simulink model "SimulateHVDC"  (R2024b)
settings: Solver=VariableStepAuto  StartTime=0.0  StopTime=Tf  FixedStep=Ti  MaxStep=Ti  RelTol=1e-6
InitFcn:
  | sim_initHVDC
StartFcn:
  | sim_initHVDC
undefined symbols (not defined in the file): CCMPC, CEMPC, DiscIntNeverNeededParam, GCC, M2C, PCC, plecs, PLL, RFT, TEB, Ti, Ts_cc, Ts_ce, Xmax, Ymax
libraries: slpidlib x5, dspstat3 x5, simulink_extras x2, spsdq0toAlphaBetaZeroLib x2, spsAlphaBetaZerotodq0Lib x2, spsabctoAlphaBetaZeroLib x2, rllib x1, deeplib x1, embmathops x1, spsabctodq0Lib x1, spsAlphaBetaZerotoabcLib x1
(part 1 of 2)
settings Model: Creator=Pablo  LastModifiedBy=Ingeniería Eléctrica
settings SolverCC: InitialStep=Ti/10  MinimalZcImpactIntegration=on

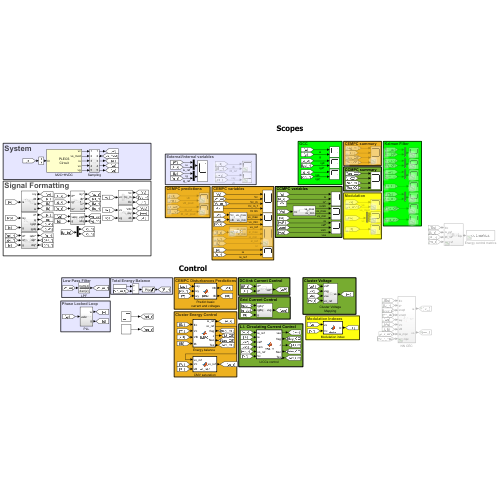
[thumbnail: Simulink's stored preview of the top-level diagram]
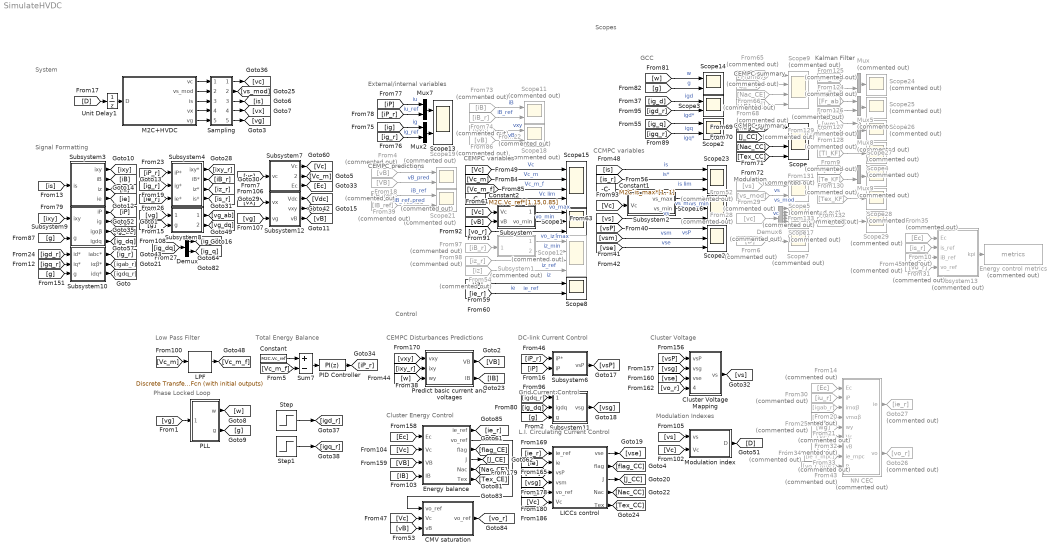
== system SimulateHVDC ==
  note: Control
  note: System
  note: Signal Formatting
  note: CCMPC summary
  note: DC-link Current Control
  note: Modulation Indexes
  note: CEMPC variables
  note: Total Energy Balance
  note: Modulation
  note: External/internal variables
  note: GCC
  note: CCMPC variables
  note: Kalman Filter
  note: CEMPC predictions
  note: CEMPC summary
  note: Low Pass Filter
  note: Cluster Energy Control
  note: CEMPC Disturbances Predictions
  note: Scopes
  note: Grid Current Control
  note: L.I. Circulating Current Control
  note: Cluster Voltage
  note: Phase Locked Loop
  CMV saturation : MATLAB Function  TreatAsAtomicUnit=on  SystemSampleTime=Ts_cc
  Cluster Voltage Mapping : Subsystem
  Constant : Constant  Value=M2C.Vc_ref  SampleTime=Ts_ce
  Constant1 : Constant  Value=M2C.is_max*[1,-1]  SampleTime=Ts_cc
  Constant2 : Constant  Value=M2C.Vc_ref*[1.15,0.85]  SampleTime=Ts_cc
  Demux : Demux  Outputs=2
  Demux6 : Demux  Commented=on  Outputs=M2C.m
  Energy balance : MATLAB Function  TreatAsAtomicUnit=on  SystemSampleTime=CEMPC.Ts
  Energy control metrics : ToWorkspace  Commented=on  VariableName=metrics  SaveFormat=Timeseries  SampleTime=-1
  From10 : From  Commented=on  GotoTag=is_r
  From124 : From  Commented=on  GotoTag=im_ab
  From125 : From  Commented=on  GotoTag=im_KF
  From126 : From  Commented=on  GotoTag=Fr_ab
  From127 : From  Commented=on  GotoTag=Fr_KF
  From128 : From  Commented=on  GotoTag=wm
  From129 : From  Commented=on  GotoTag=wm_KF
  From130 : From  Commented=on  GotoTag=Te
  From131 : From  Commented=on  GotoTag=Te_KF
  From132 : From  Commented=on  GotoTag=Tex_KF
  From133 : From  Commented=on  GotoTag=NIS_KF
  From14 : From  Commented=on  GotoTag=Ec
  From18 : From  Commented=on  GotoTag=VB
  From20 : From  Commented=on  GotoTag=igab_r
  From21 : From  Commented=on  GotoTag=vm_ab
  From22 : From  Commented=on  GotoTag=vB
  From25 : From  Commented=on  GotoTag=wg
  From28 : From  Commented=on  GotoTag=vc
  From29 : From  Commented=on  GotoTag=vs
  From30 : From  Commented=on  GotoTag=iu_r
  From31 : From  Commented=on  GotoTag=iB_r
  From32 : From  Commented=on  GotoTag=Vc
  From33 : From  Commented=on  GotoTag=vB
  From34 : From  Commented=on  GotoTag=ie_r_mpc
  From35 : From  Commented=on  GotoTag=Ec
  From36 : From  Commented=on  GotoTag=IB_ref
  From39 : From  Commented=on  GotoTag=iB_ref
  From4 : From  Commented=on  GotoTag=vB
  From43 : From  Commented=on  GotoTag=vo_r_mpc
  From45 : From  Commented=on  GotoTag=vo_r
  From52 : From  Commented=on  GotoTag=vs_mod
  From54 : From  Commented=on  GotoTag=iz
  From6 : From  Commented=on  GotoTag=D
  From65 : From  Commented=on  GotoTag=flag_CE
  From66 : From  Commented=on  GotoTag=J_CE
  From67 : From  Commented=on  GotoTag=Nac_CE
  From68 : From  Commented=on  GotoTag=Tex_CE
  From73 : From  Commented=on  GotoTag=iB
  From74 : From  Commented=on  GotoTag=iB_r
  From86 : From  Commented=on  GotoTag=vxy
  From9 : From  Commented=on  GotoTag=Tl_KF
  From97 : From  Commented=on  GotoTag=iB_r
  From98 : From  Commented=on  GotoTag=iz_r
  Goto26 : Goto  Commented=on  GotoTag=vo_r
  Goto27 : Goto  Commented=on  GotoTag=ie_r
  LICCs control : MATLAB Function  TreatAsAtomicUnit=on  SystemSampleTime=CCMPC.Ts
  LPF : simulink_extras/Additional Discrete/Discrete Transfer Fcn (with initial outputs)  N=[TEB.b1 TEB.b0]  D=[TEB.a1 TEB.a0]  U0=M2C.Vc_ref  Y0=M2C.Vc_ref  TS=TEB.Ts
  M2C+HVDC : Subsystem  LoadFcn=plecs('sl', 200);  InitFcn=plecs('sl', 214);  StartFcn=plecs('sl', 208);  StopFcn=plecs('sl', 209);  mask(PlecsCircuit){PLECSData=<binary blob, 24188 chars, not shown>}
      mask prompts: PLECSData "PLECS Data (Do not delete or modify!)"
      mask init:
      | % PLACE CUSTOM INITIALIZATIONS ABOVE
      | % DO NOT REMOVE
      | plecs('sl', 215);
      | % DO NOT REMOVE
      settings: CopyFcn=plecs('sl', 203);  DeleteFcn=plecs('sl', 205);  UndoDeleteFcn=plecs('sl', 206);  PreSaveFcn=plecs('sl', 211);  PostSaveFcn=plecs('sl', 201);  NameChangeFcn=plecs('sl', 210);  DestroyFcn=plecs('sl', 207);  PreCopyFcn=plecs('sl', 216);  OpenFcn=plecs('sl', 202);  ErrorFcn=plerrorfcn
      mask Help: eval('plecs(''help'', ''qthelp:///creatingacircuit.html'')')
      mask Display: disp('PLECS\nCircuit')
  Modulation index : MATLAB Function  TreatAsAtomicUnit=on  SystemSampleTime=CCMPC.Ts
  Mux : Mux  Commented=on  Inputs=[2; 2]
  Mux2 : Mux  Inputs=[3; 3]
  Mux5 : Mux  Commented=on  Inputs=[2; 2]
  Mux7 : Mux  Inputs=2
  Mux8 : Mux  Commented=on  Inputs=2
  Mux9 : Mux  Commented=on  Inputs=2
  NN CEC : Subsystem  Commented=on
  PID Controller : slpidlib/PID Controller  Controller=PI  Form=Parallel  TimeDomain=Discrete-time  UseExternalTs=off  SampleTime=TEB.Ts  IntegratorMethod=Forward Euler  FilterMethod=Forward Euler  ControllerParametersSource=internal  P=TEB.kp  I=TEB.ki  UseKiTs=off  D=0  UseExternalDerivativeSource=off  N=100  UseFilter=on  TunerSelectOption=Transfer Function Based (PID Tuner App)  InitialConditionSource=internal  InitialConditionForIntegrator=0  InitialConditionForFilter=0  DifferentiatorICPrevScaledInput=0  ExternalReset=none  TrackingMode=off  Kt=1  LimitOutput=on  SatLimitsSource=internal  UpperSaturationLimit=TEB.u_max  LowerSaturationLimit=TEB.u_min  LinearizeAsGain=on  AntiWindupMode=clamping  Kb=TEB.kp  LimitIntegrator=off  UpperIntegratorSaturationLimit=inf  LowerIntegratorSaturationLimit=-inf  POutMin=[]  POutMax=[]  IOutMin=[]  IOutMax=[]  DOutMin=[]  DOutMax=[]  NOutMin=[]  NOutMax=[]  SumOutMin=[]  SumOutMax=[]  SaturationOutMin=[]  SaturationOutMax=[]  PParamMin=[]  PParamMax=[]  IParamMin=[]  IParamMax=[]  DParamMin=[]  DParamMax=[]  NParamMin=[]  NParamMax=[]  KbParamMin=[]  KbParamMax=[]  KtParamMin=[]  KtParamMax=[]  KbOutMin=[]  KbOutMax=[]  KtOutMin=[]  KtOutMax=[]  IntegratorOutMin=[]  IntegratorOutMax=[]  FilterOutMin=[]  FilterOutMax=[]  SumI1OutMin=[]  SumI1OutMax=[]  SumI2OutMin=[]  SumI2OutMax=[]  SumI3OutMin=[]  SumI3OutMax=[]  SumI4OutMin=[]  SumI4OutMax=[]  SumDOutMin=[]  SumDOutMax=[]  DifferentiatorOutMin=[]  DifferentiatorOutMax=[]  FilterDiffOutCoefMin=[]  FilterDiffOutCoefMax=[]  ReciprocalOutMin=[]  ReciprocalOutMax=[]  SumDenOutMin=[]  SumDenOutMax=[]  SumNumOutMin=[]  SumNumOutMax=[]  DivideOutMin=[]  DivideOutMax=[]  UdiffTsProdOutMin=[]  UdiffTsProdOutMax=[]  NTsProdOutMin=[]  NTsProdOutMax=[]  UintegralTsProdOutMin=[]  UintegralTsProdOutMax=[]  UngainTsProdOutMin=[]  UngainTsProdOutMax=[]  ClampingZeroOutDataTypeStr=Inherit: Inherit via back propagation  ClampingZeroOutMin=[]  ClampingZeroOutMax=[]  FilterDenConstantOutDataTypeStr=Inherit: Inherit via back propagation  FilterDenConstantOutMin=[]  FilterDenConstantOutMax=[]  PCopyOutDataTypeStr=Inherit: Inherit via back propagation  PCopyOutMin=[]  PCopyOutMax=[]  NCopyOutDataTypeStr=Inherit: Inherit via back propagation  NCopyOutMin=[]  NCopyOutMax=[]  IntegratorContinuousStateAttributes=''  IntegratorStateMustResolveToSignalObject=off  IntegratorRTWStateStorageClass=Auto  FilterContinuousStateAttributes=''  FilterStateMustResolveToSignalObject=off  FilterRTWStateStorageClass=Auto  ParallelPVariant=InternalParameters  IdealPVariant=Disabled  IVariant=InternalParameters  DVariant=Disabled  IntegratorVariant=Discrete  SatVariant=Enabled  AWVariant=DiscClampingParallel  PCopyVariant=Disabled  TRVariant=Disabled  FdbkBlocksVariant=Forward  IdealPFdbkVariant=Disabled  SatFdbkVariant=Disabled  DerivativeFilterVariant=Disabled  NVariant=Disabled  NCopyVariant=Disabled_SignalSpec  FilterICVariant=Disabled  IntegratorICVariant=InternalICs  ExternalResetVariant=Disabled  TRSumVariant=Passthrough  SumFdbkVariant=Disabled  SumVariant=Sum_PI  TsampFilterVariant=InternalTs  TsampNgainVariant=Passthrough  TsampIntegralVariant=Disabled_SignalSpec  ExternalSaturationOutDataTypeStr=Inherit: Same as second input  DerivativeSourceVariant=Disabled  PreIntVariant=InternalPreInt
  PLL : Subsystem
  Predict basic current and voltages : MATLAB Function  TreatAsAtomicUnit=on  SystemSampleTime=CEMPC.Ts
  Sampling : Subsystem
  Scope : Scope  NumInputPorts=4
  Scope{1,16,20,23} (4 alike) : Scope  NumInputPorts=3
  Scope{5,11,18..19,21} (5 alike) : Scope  Commented=on  NumInputPorts=2
  Scope12 : Scope  Commented=on  NumInputPorts=4
  Scope{2..3,8,13..14} (5 alike) : Scope  NumInputPorts=2
  Scope15 : Scope  NumInputPorts=4
  Scope17 : Scope  Commented=on  NumInputPorts=6
  Scope{4,7,24..29} (8 alike) : Scope  Commented=on
  Scope9 : Scope  Commented=on  NumInputPorts=4
  Step : Step  After=1000  SampleTime=Ts_ce
  Step1 : Step  Time=2  After=200  SampleTime=Ts_ce
  Subsystem : Subsystem
  Subsystem1 : Subsystem  Commented=on
  Subsystem10 : Subsystem
  Subsystem11 : Subsystem
  Subsystem12 : Subsystem
  Subsystem13 : Subsystem  Commented=on
  Subsystem2 : Subsystem
  Subsystem3 : Subsystem
  Subsystem4 : Subsystem
  Subsystem6 : Subsystem
  Subsystem7 : Subsystem
  Subsystem8 : Subsystem
  Subsystem9 : Subsystem
  Sum7 : Sum  Inputs=+-
  Unit Delay1 : UnitDelay  InitialCondition=zeros(6, 1)  SampleTime=Ti  HasFrameUpgradeWarning=on
  wires:
  Sum7/1 -> PID Controller/1
  Subsystem3/2(iB) -> [iB]
  [Vc_m] -> Scope15/2  "Vc_m"
  From125/1 -> Mux/2
  [iP_r] -> Subsystem4/1(iP*)
  Subsystem7/3(Ec) -> [Ec]
  Mux7/1 -> Scope13/1
  Subsystem9/4(igdq) -> [ig_dq]
  Demux6/6 -> Scope17/6
  [is_r] -> Scope23/2  "is*"
  From130/1 -> Mux9/1
  [Vc] -> Subsystem2/1(Vc)
  Subsystem10/2(iαβ*) -> [igab_r]
  Subsystem/2(vo_min) -> Scope1/2  "vo_min"
  From127/1 -> Mux5/2
  [igd_r] -> Subsystem10/1(id*)
  [Vc] -> Scope15/1  "Vc"
  From29/1 -> Scope5/1  "vs"
  [igd_r] -> Scope3/2  "igd*"
  [D] -> Unit Delay1/1
  Subsystem12/1(Vdc) -> [Vdc]
  Demux6/2 -> Scope17/2
  From36/1 -> Scope21/2  "iB_ref_pred"
  Subsystem4/3(iz*) -> [iz_r]
  Demux6/1 -> Scope17/1
  [igq_r] -> Subsystem10/2(iq*)
  Subsystem7/1(Vc) -> [Vc]
  [iP] -> Mux7/1  "iu"
  Subsystem3/3(iz) -> [iz]
  Mux9/1 -> Scope27/1
  From97/1 -> Subsystem1/1(iB_ref)
  [g] -> Subsystem8/2(g)
  Subsystem2/1(vs_max) -> Scope16/1  "vs_max"
  Subsystem4/4(is*) -> [is_r]
  From133/1 -> Scope29/1
  Subsystem9/1(iP) -> [iP]
  [ixy] -> Subsystem9/1(ixy)
  Subsystem10/3(idq*) -> [igdq_r]
  From126/1 -> Mux5/1
  [Vc_m] -> LPF/1
  Subsystem7/2(Vc_m) -> [Vc_m]
  Subsystem3/1(ixy) -> [ixy]
  Subsystem2/2(vs_min) -> Scope16/2  "vs_min"
  Demux6/3 -> Scope17/3
  From4/1 -> Scope19/1  "vB"
  [Vc_m_f] -> Scope15/3  "Vc_m_f"
  M2C+HVDC/2(vs_mod) -> Sampling/2(In2)
  From18/1 -> Scope19/2  "vB_pred"
  From67/1 -> Scope9/3
  [ig] -> Mux2/1  "ig"
  Sampling/3(Out3) -> [is]
  Sampling/4(Out4) -> [vx]
  [vc] -> Subsystem7/1(vc)
  [flag_CC] -> Scope/1
  Subsystem10/1(iabc*) -> [ig_r]
  [J_CC] -> Scope/2
  Subsystem4/2(iB*) -> [iB_r]
  [ig_r] -> Mux2/2  "ig_ref"
  Demux6/4 -> Scope17/4
  Sampling/1(Out1) -> [vc]
  [g] -> Subsystem10/3(g)
  Subsystem/1(vo_max) -> Scope1/1  "vo_max"
  LPF/1 -> [Vc_m_f]
  From86/1 -> Scope18/1  "vxy"
  [vx] -> Subsystem12/1(vx)
  Subsystem8/2(vdq) -> [vg_dq]
  [ie_r] -> Scope8/2  "ie_ref"
  Subsystem9/3(igαβ) -> [ig_ab]
  Predict basic current and voltages/1(VB) -> [VB]
  [is] -> Subsystem3/1(is)
  [iP_r] -> Mux7/2  "iu_ref"
  [vg] -> Subsystem12/2(vg)
  [vo_r] -> Scope1/3  "vo_ref"
  [vg] -> Subsystem8/1(vabc)
  [Nac_CC] -> Scope/3
  [vB] -> Subsystem/2(vB)
  Mux2/1 -> Scope13/2
  From66/1 -> Scope9/2
  Demux/2 -> [ig_q]
  [ig_dq] -> Demux/1
  From73/1 -> Scope11/1  "iB"
  From65/1 -> Scope9/1
  Mux5/1 -> Scope25/1
  From128/1 -> Mux8/1
  [Vc] -> Subsystem/1(Vc)
  Subsystem3/4(ie) -> [ie]
  [vxy] -> Predict basic current and voltages/1(vxy)
  Unit Delay1/1 -> M2C+HVDC/1(D)
  Constant/1 -> Sum7/1
  [ie_r] -> Subsystem4/3(ie*)
  From6/1 -> Scope7/1
  [is] -> Scope23/1  "is"
  [ig_r] -> Subsystem4/2(ig*)
  Subsystem12/3(vB) -> [vB]
  Subsystem9/2(ig) -> [ig]
  Subsystem8/1(vαβ) -> [vg_ab]
  [Tex_CC] -> Scope/4
  From39/1 -> Scope21/1  "iB_ref"
  [vs] -> Scope16/3  "vs"
  Subsystem1/2(iz_min) -> Scope12/2  "iz_min"
  From52/1 -> Scope5/2  "vs_mod"
  Predict basic current and voltages/2(IB) -> [IB]
  Demux6/5 -> Scope17/5
  From28/1 -> Demux6/1  "vc"
  [w] -> Predict basic current and voltages/3(wy)
  Subsystem1/1(iz_max) -> Scope12/1  "iz_max"
  M2C+HVDC/1(vc) -> Sampling/1(In1)
  Demux/1 -> [ig_d]
  [ixy_r] -> Predict basic current and voltages/2(ixy)
  From129/1 -> Mux8/2
  From68/1 -> Scope9/4
  Mux8/1 -> Scope26/1
  From131/1 -> Mux9/2
  From22/1 -> Scope18/2  "vB"
  Sampling/2(Out2) -> [vs_mod]
  Subsystem4/1(ixy*) -> [ixy_r]
  [g] -> Subsystem9/2(g)
  [ig_d] -> Scope3/1  "igd"
  Mux/1 -> Scope24/1
  From74/1 -> Scope11/2  "iB_ref"
  From98/1 -> Scope12/3  "iz_ref"
  From132/1 -> Scope28/1
  [ie] -> Scope8/1  "ie"
  From124/1 -> Mux/1
  [vs] -> Modulation index/1(vs)
  [Vc] -> Modulation index/2(Vc)
  Modulation index/1(D) -> [D]
  Energy balance/4(J) -> [J_CE]
  Energy balance/5(Nac) -> [Nac_CE]
  Energy balance/6(Tex) -> [Tex_CE]
  Energy balance/1(ie_ref) -> [ie_r]
  [Ec] -> Energy balance/1(Ec)
  [Vc] -> Energy balance/2(Vc)
  [VB] -> Energy balance/3(VB)
  [IB] -> Energy balance/4(IB)
  [ie_r] -> LICCs control/1(ie_ref)
  [ie] -> LICCs control/2(ie)
  [vsg] -> LICCs control/4(vsm)
  [vsP] -> LICCs control/3(vsP)
  [vo_r] -> LICCs control/5(vo_ref)
  [Vc] -> LICCs control/6(Vc)
  LICCs control/1(vse) -> [vse]
  LICCs control/2(flag) -> [flag_CC]
  LICCs control/3(J) -> [J_CC]
  LICCs control/4(Nac) -> [Nac_CC]
  LICCs control/5(Tex) -> [Tex_CC]
  [vsP] -> Cluster Voltage Mapping/1(vsP)
  [vse] -> Cluster Voltage Mapping/3(vse)
  [vo_r] -> Cluster Voltage Mapping/4(vo_ref)
  Cluster Voltage Mapping/1(vs) -> [vs]
  Subsystem12/2(vxy) -> [vxy]
  [w] -> Scope14/1  "w"
  [g] -> Scope14/2  "g"
  [vsm] -> Scope20/2  "vsm"
  [vsP] -> Scope20/1  "vsP"
  [vse] -> Scope20/3  "vse"
  [Vc_m_f] -> Sum7/2
  [iP_r] -> Subsystem6/1(iP*)
  [iP] -> Subsystem6/2(iP)
  Subsystem6/1(vsP) -> [vsP]
  [igdq_r] -> Subsystem11/1(igdq*)
  [ig_dq] -> Subsystem11/2(igdq)
  Subsystem11/1(vsg) -> [vsg]
  From14/1 -> NN CEC/1(Ec)
  Constant1/1 -> Scope23/3  "is lim"
  Constant2/1 -> Scope15/4  "Vc lim"
  From30/1 -> NN CEC/2(iP)
  From20/1 -> NN CEC/3(imαβ)
  From21/1 -> NN CEC/4(vmαβ)
  From25/1 -> NN CEC/5(wy)
  NN CEC/1(ie) -> Goto27/1
  NN CEC/2(vo) -> Goto26/1
  Energy balance/3(flag) -> [flag_CE]
  From32/1 -> NN CEC/6(Vc)
  From33/1 -> NN CEC/7(vB)
  From54/1 -> Scope12/4  "iz"
  From9/1 -> Scope4/1
  [vsg] -> Cluster Voltage Mapping/2(vsg)
  From35/1 -> Subsystem13/1(Ec)
  From10/1 -> Subsystem13/2(is_ref)
  From31/1 -> Subsystem13/3(iB_ref)
  From45/1 -> Subsystem13/4(vo_ref)
  Subsystem13/1(kpi) -> Energy control metrics/1
  From34/1 -> NN CEC/8(ie_mpc)
  From43/1 -> NN CEC/9(vo_mpc)
  CMV saturation/1(vo_ref) -> [vo_r]
  [Vc] -> CMV saturation/2(Vc)
  [vB] -> CMV saturation/3(vB)
  Energy balance/2(vo_ref) -> CMV saturation/1("vo_ref ")
  M2C+HVDC/3(is) -> Sampling/3(In3)
  M2C+HVDC/4(vx) -> Sampling/4(In4)
  M2C+HVDC/5(vg) -> Sampling/5(In5)
  Sampling/5(Out5) -> [vg]
  PLL/1(w) -> [w]
  PLL/2(g) -> [g]
  [vg] -> PLL/1(vabc)
  Step/1 -> [igd_r]
  Step1/1 -> [igq_r]
  [g] -> Subsystem11/3(g)
  [ig_q] -> Scope2/1  "igq"
  [igq_r] -> Scope2/2  "igq*"
  PID Controller/1 -> [iP_r]

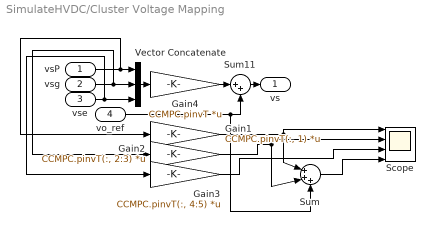
== system SimulateHVDC/Cluster Voltage Mapping ==
  vsP : Inport
  vsg : Inport  Port=2
  vse : Inport  Port=3
  vo_ref : Inport  Port=4
  Gain1 : Gain  Gain=CCMPC.pinvT(:, 1)  Multiplication=Matrix(K*u) (u vector)
  Gain2 : Gain  Gain=CCMPC.pinvT(:, 2:3)  Multiplication=Matrix(K*u) (u vector)
  Gain3 : Gain  Gain=CCMPC.pinvT(:, 4:5)  Multiplication=Matrix(K*u) (u vector)
  Gain4 : Gain  Gain=CCMPC.pinvT  Multiplication=Matrix(K*u) (u vector)
  Scope : Scope  NumInputPorts=4
  Sum : Sum  Inputs=|+++
  Sum11 : Sum  Inputs=|++
  Vector Concatenate : Concatenate  NumInputs=3
  vs : Outport
  wires:
  Gain4/1 -> Sum11/1
  Vector Concatenate/1 -> Gain4/1
  vsg/1 -> Gain2/1, Vector Concatenate/2
  vsP/1 -> Gain1/1, Vector Concatenate/1
  vo_ref/1 -> Sum/3, Sum11/2
  vse/1 -> Vector Concatenate/3, Gain3/1
  Sum11/1 -> vs/1
  Gain1/1 -> Sum/1, Scope/1
  Gain2/1 -> Sum/2, Scope/2
  Gain3/1 -> Scope/3
  Sum/1 -> Scope/4

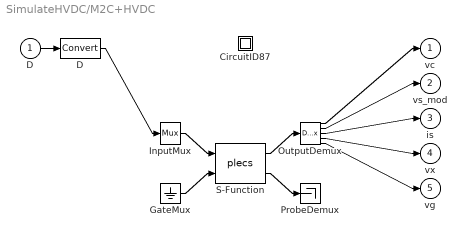
== system SimulateHVDC/M2C+HVDC ==
  D : Inport  PortDimensions=6
  " CircuitID87 " : Subsystem
  " D " : DataTypeConversion
  " GateMux " : Ground
  " InputMux " : Mux  Inputs=[ 6 ]
  " OutputDemux " : Demux  Outputs=[ 24 6 6 2 3 ]
  " ProbeDemux " : Terminator
  " S-Function " : S-Function  FunctionName=plecs  SFunctionDeploymentMode=off  EnableBusSupport=off
  vc : Outport  PortDimensions=24
  vs_mod : Outport  Port=2  PortDimensions=6
  is : Outport  Port=3  PortDimensions=6
  vx : Outport  Port=4  PortDimensions=2
  vg : Outport  Port=5  PortDimensions=3
  wires:
  " InputMux "/1 -> " S-Function "/1
  " GateMux "/1 -> " S-Function "/2
  " S-Function "/1 -> " OutputDemux "/1
  " S-Function "/2 -> " ProbeDemux "/1
  D/1 -> " D "/1
  " D "/1 -> " InputMux "/1
  " OutputDemux "/1 -> vc/1
  " OutputDemux "/2 -> vs_mod/1
  " OutputDemux "/3 -> is/1
  " OutputDemux "/4 -> vx/1
  " OutputDemux "/5 -> vg/1

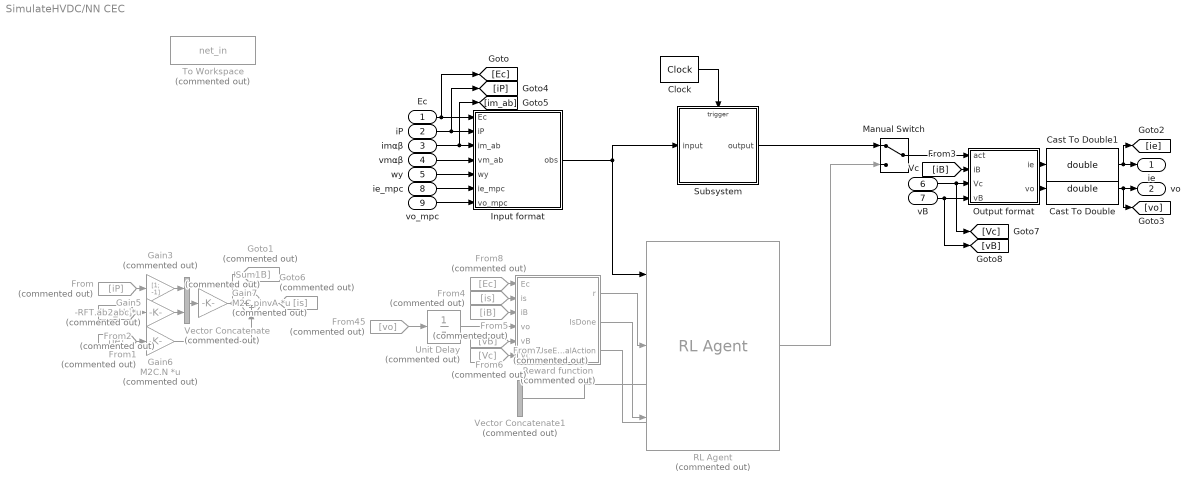
== system SimulateHVDC/NN CEC ==
  Ec : Inport
  iP : Inport  Port=2
  imαβ : Inport  Port=3
  vmαβ : Inport  Port=4
  wy : Inport  Port=5
  Vc : Inport  Port=6
  vB : Inport  Port=7
  ie_mpc : Inport  Port=8
  vo_mpc : Inport  Port=9
  Cast To Double : DataTypeConversion  OutDataTypeStr=double  SaturateOnIntegerOverflow=off  RndMeth=Floor
  Cast To Double1 : DataTypeConversion  OutDataTypeStr=double  SaturateOnIntegerOverflow=off  RndMeth=Floor
  Clock : simulink_extras/Flip Flops/Clock  period=Ts_ce
  From : From  Commented=on  GotoTag=iP
  From1 : From  Commented=on  GotoTag=ie
  From2 : From  Commented=on  GotoTag=im_ab
  From4 : From  Commented=on  GotoTag=is
  From45 : From  Commented=on  GotoTag=vo
  From5 : From  Commented=on  GotoTag=iB
  From6 : From  Commented=on  GotoTag=vB
  From7 : From  Commented=on  GotoTag=Vc
  From8 : From  Commented=on  GotoTag=Ec
  Gain3 : Gain  Commented=on  Gain=[1; -1]
  Gain5 : Gain  Commented=on  Gain=-RFT.ab2abc  Multiplication=Matrix(K*u) (u vector)
  Gain6 : Gain  Commented=on  Gain=M2C.N  Multiplication=Matrix(K*u) (u vector)
  Gain7 : Gain  Commented=on  Gain=M2C.pinvA  Multiplication=Matrix(K*u) (u vector)
  Goto1 : Goto  Commented=on  GotoTag=iB
  Goto6 : Goto  Commented=on  GotoTag=is
  Input format : MATLAB Function  TreatAsAtomicUnit=on  SystemSampleTime=Ts_ce
  Manual Switch : ManualSwitch
  Output format : MATLAB Function  TreatAsAtomicUnit=on  SystemSampleTime=Ts_ce
  RL Agent : rllib/RL Agent  Commented=on  Agent=agent  ExternalActionAsInput=off  ProvideLastAction=off  ProvideCumRwd=off  TreatAsDirectFeedthrough=on  UseStrictObservationDataTypes=off
  Reward function : MATLAB Function  Commented=on  TreatAsAtomicUnit=on  SystemSampleTime=Ts_ce
  Subsystem : Subsystem
  Sum1 : Sum  Commented=on  Inputs=|++
  To Workspace : ToWorkspace  Commented=on  VariableName=net_in  SaveFormat=Timeseries  SampleTime=Ts_ce
  Unit Delay : UnitDelay  Commented=on  SampleTime=Ts_ce  HasFrameUpgradeWarning=on
  Vector Concatenate : Concatenate  Commented=on
  Vector Concatenate1 : Concatenate  Commented=on
  ie : Outport
  vo : Outport  Port=2
  wires:
  Input format/1(obs) -> Subsystem/1(input), RL Agent/1
  iP/1 -> [iP], Input format/2(iP)
  Cast To Double1/1 -> [ie], ie/1
  vB/1 -> Output format/4(vB), [vB]
  Vector Concatenate/1 -> Gain7/1
  Gain3/1 -> Vector Concatenate/1
  Vc/1 -> [Vc], Output format/3(Vc)
  imαβ/1 -> [im_ab], Input format/3(im_ab)
  Output format/2(vo) -> Cast To Double/1
  Manual Switch/1 -> Output format/1(act)
  Gain5/1 -> Vector Concatenate/2
  Reward function/1(r) -> RL Agent/2
  Output format/1(ie) -> Cast To Double1/1
  Gain7/1 -> Sum1/1, Goto1/1
  wy/1 -> Input format/5(wy)
  From2/1 -> Gain5/1
  [iB] -> Output format/2(iB)
  RL Agent/1 -> Manual Switch/2
  Ec/1 -> [Ec], Input format/1(Ec)
  Gain6/1 -> Sum1/2
  From1/1 -> Gain6/1
  vmαβ/1 -> Input format/4(vm_ab)
  Cast To Double/1 -> [vo], vo/1
  From/1 -> Gain3/1
  Subsystem/1(output) -> Manual Switch/1
  Clock/1 -> Subsystem/Trigger
  Sum1/1 -> Goto6/1
  From8/1 -> Reward function/1(Ec)
  From4/1 -> Reward function/2(is)
  From45/1 -> Unit Delay/1
  From5/1 -> Reward function/3(iB)
  From6/1 -> Reward function/5(vB)
  From7/1 -> Reward function/6(Vc)
  Reward function/2(IsDone) -> RL Agent/3
  ? -> Vector Concatenate1/2
  ? -> Vector Concatenate1/1
  Vector Concatenate1/1 -> ?
  Reward function/3(UseExternalAction) -> ?
  Unit Delay/1 -> Reward function/4(vo)
  ie_mpc/1 -> Input format/6(ie_mpc)
  vo_mpc/1 -> Input format/7(vo_mpc)

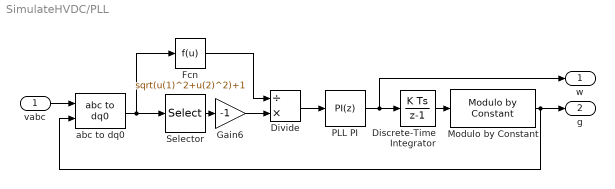
== system SimulateHVDC/PLL ==
  vabc : Inport
  Discrete-Time Integrator : DiscreteIntegrator  SampleTime=PLL.Ts  ICPrevOutput=DiscIntNeverNeededParam  ICPrevScaledInput=DiscIntNeverNeededParam
  Divide : Product  Inputs=/*
  Fcn : Fcn  Expr=sqrt(u(1)^2+u(2)^2)+1
  Gain6 : Gain  Gain=-1
  Modulo by Constant : embmathops/Modulo by Constant  Denominator=2*pi  SimulateUsing=Code generation
      settings: LibrarySourceBlock=embeddedMathLib/Modulo by Constant
  PLL PI : slpidlib/PID Controller  Controller=PI  Form=Parallel  TimeDomain=Discrete-time  UseExternalTs=off  SampleTime=PLL.Ts  IntegratorMethod=Forward Euler  FilterMethod=Forward Euler  ControllerParametersSource=internal  P=PLL.kp  I=PLL.ki  UseKiTs=off  D=0  UseExternalDerivativeSource=off  N=100  UseFilter=on  TunerSelectOption=Transfer Function Based (PID Tuner App)  InitialConditionSource=internal  InitialConditionForIntegrator=100*pi  InitialConditionForFilter=0  DifferentiatorICPrevScaledInput=0  ExternalReset=none  TrackingMode=off  Kt=1  LimitOutput=off  SatLimitsSource=internal  UpperSaturationLimit=inf  LowerSaturationLimit=-inf  LinearizeAsGain=on  AntiWindupMode=none  Kb=1  LimitIntegrator=off  UpperIntegratorSaturationLimit=inf  LowerIntegratorSaturationLimit=-inf  POutMin=[]  POutMax=[]  IOutMin=[]  IOutMax=[]  DOutMin=[]  DOutMax=[]  NOutMin=[]  NOutMax=[]  SumOutMin=[]  SumOutMax=[]  SaturationOutMin=[]  SaturationOutMax=[]  PParamMin=[]  PParamMax=[]  IParamMin=[]  IParamMax=[]  DParamMin=[]  DParamMax=[]  NParamMin=[]  NParamMax=[]  KbParamMin=[]  KbParamMax=[]  KtParamMin=[]  KtParamMax=[]  KbOutMin=[]  KbOutMax=[]  KtOutMin=[]  KtOutMax=[]  IntegratorOutMin=[]  IntegratorOutMax=[]  FilterOutMin=[]  FilterOutMax=[]  SumI1OutMin=[]  SumI1OutMax=[]  SumI2OutMin=[]  SumI2OutMax=[]  SumI3OutMin=[]  SumI3OutMax=[]  SumI4OutMin=[]  SumI4OutMax=[]  SumDOutMin=[]  SumDOutMax=[]  DifferentiatorOutMin=[]  DifferentiatorOutMax=[]  FilterDiffOutCoefMin=[]  FilterDiffOutCoefMax=[]  ReciprocalOutMin=[]  ReciprocalOutMax=[]  SumDenOutMin=[]  SumDenOutMax=[]  SumNumOutMin=[]  SumNumOutMax=[]  DivideOutMin=[]  DivideOutMax=[]  UdiffTsProdOutMin=[]  UdiffTsProdOutMax=[]  NTsProdOutMin=[]  NTsProdOutMax=[]  UintegralTsProdOutMin=[]  UintegralTsProdOutMax=[]  UngainTsProdOutMin=[]  UngainTsProdOutMax=[]  ClampingZeroOutDataTypeStr=Inherit: Inherit via back propagation  ClampingZeroOutMin=[]  ClampingZeroOutMax=[]  FilterDenConstantOutDataTypeStr=Inherit: Inherit via back propagation  FilterDenConstantOutMin=[]  FilterDenConstantOutMax=[]  PCopyOutDataTypeStr=Inherit: Inherit via back propagation  PCopyOutMin=[]  PCopyOutMax=[]  NCopyOutDataTypeStr=Inherit: Inherit via back propagation  NCopyOutMin=[]  NCopyOutMax=[]  IntegratorContinuousStateAttributes=''  IntegratorStateMustResolveToSignalObject=off  IntegratorRTWStateStorageClass=Auto  FilterContinuousStateAttributes=''  FilterStateMustResolveToSignalObject=off  FilterRTWStateStorageClass=Auto  ParallelPVariant=InternalParameters  IdealPVariant=Disabled  IVariant=InternalParameters  DVariant=Disabled  IntegratorVariant=Discrete  SatVariant=Disabled  AWVariant=Passthrough  PCopyVariant=Disabled  TRVariant=Disabled  FdbkBlocksVariant=Forward  IdealPFdbkVariant=Disabled  SatFdbkVariant=Disabled  DerivativeFilterVariant=Disabled  NVariant=Disabled  NCopyVariant=Disabled_SignalSpec  FilterICVariant=Disabled  IntegratorICVariant=InternalICs  ExternalResetVariant=Disabled  TRSumVariant=Passthrough  SumFdbkVariant=Disabled  SumVariant=Sum_PI  TsampFilterVariant=InternalTs  TsampNgainVariant=Passthrough  TsampIntegralVariant=Disabled_SignalSpec  ExternalSaturationOutDataTypeStr=Inherit: Same as second input  DerivativeSourceVariant=Disabled  PreIntVariant=InternalPreInt
  Selector : Selector  InputPortWidth=3  IndexOptions=Index vector (dialog)  Indices=[2]  OutputSizes=1
  abc to dq0 : spsabctodq0Lib/abc to dq0  Alignment=Aligned with phase A axis
  w : Outport
  g : Outport  Port=2
  wires:
  Discrete-Time Integrator/1 -> Modulo by Constant/1
  vabc/1 -> abc to dq0/1
  Modulo by Constant/1 -> g/1, abc to dq0/2
  abc to dq0/1 -> Fcn/1, Selector/1
  Selector/1 -> Gain6/1
  PLL PI/1 -> w/1, Discrete-Time Integrator/1
  Fcn/1 -> Divide/1
  Gain6/1 -> Divide/2
  Divide/1 -> PLL PI/1

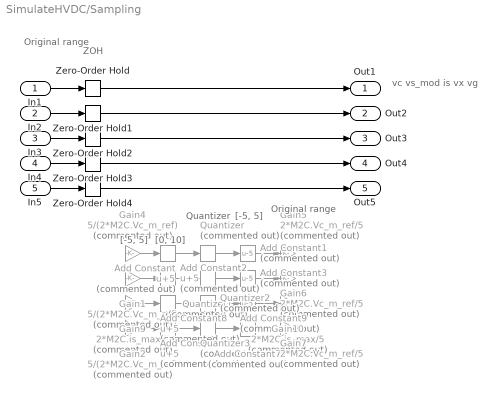
== system SimulateHVDC/Sampling ==
  note: ZOH
  note: vc
      |
      | vs_mod
      |
      | is
      |
      | vx
      |
      | vg
  note: Original
      | range
  note: Quantizer
  note: Original
      | range
  note: [-5, 5]
  note: [0, 10]
  note: [-5, 5]
  In1 : Inport
  In2 : Inport  Port=2
  In3 : Inport  Port=3
  In4 : Inport  Port=4
  In5 : Inport  Port=5
  Add Constant{,2,6,8} (4 alike) : Bias  Commented=on  Bias=5  SaturateOnIntegerOverflow=off
  Add Constant{1,3,7,9} (4 alike) : Bias  Commented=on  Bias=-5  SaturateOnIntegerOverflow=off
  Gain1 : Gain  Commented=on  Gain=5/(2*M2C.Vc_m_ref)
  Gain10 : Gain  Commented=on  Gain=2*M2C.is_max/5
  Gain2 : Gain  Commented=on  Gain=5/(2*M2C.Vc_m_ref)
  Gain4 : Gain  Commented=on  Gain=5/(2*M2C.Vc_m_ref)
  Gain5 : Gain  Commented=on  Gain=2*M2C.Vc_m_ref/5
  Gain6 : Gain  Commented=on  Gain=2*M2C.Vc_m_ref/5
  Gain7 : Gain  Commented=on  Gain=2*M2C.Vc_m_ref/5
  Gain9 : Gain  Commented=on  Gain=2*M2C.is_max/5
  Quantizer{,1..3} (4 alike) : Quantizer  Commented=on  QuantizationInterval=10/(2^12-1)
  Zero-Order Hold{,1..4} (5 alike) : ZeroOrderHold  SampleTime=CCMPC.Ts
  Out1 : Outport
  Out2 : Outport  Port=2
  Out3 : Outport  Port=3
  Out4 : Outport  Port=4
  Out5 : Outport  Port=5
  wires:
  In4/1 -> Zero-Order Hold3/1
  In3/1 -> Zero-Order Hold2/1
  In2/1 -> Zero-Order Hold1/1
  In1/1 -> Zero-Order Hold/1
  Add Constant8/1 -> Quantizer2/1
  Quantizer1/1 -> Add Constant3/1
  Add Constant2/1 -> Quantizer1/1
  Add Constant6/1 -> Quantizer3/1
  Quantizer3/1 -> Add Constant7/1
  Gain1/1 -> Add Constant2/1
  Quantizer2/1 -> Add Constant9/1
  Gain9/1 -> Add Constant8/1
  Quantizer/1 -> Add Constant1/1
  Add Constant7/1 -> Gain7/1
  Gain4/1 -> Add Constant/1
  Add Constant/1 -> Quantizer/1
  Add Constant1/1 -> Gain5/1
  Add Constant3/1 -> Gain6/1
  Gain2/1 -> Add Constant6/1
  Add Constant9/1 -> Gain10/1
  Zero-Order Hold2/1 -> Out3/1
  Zero-Order Hold/1 -> Out1/1
  Zero-Order Hold1/1 -> Out2/1
  Zero-Order Hold3/1 -> Out4/1
  In5/1 -> Zero-Order Hold4/1
  Zero-Order Hold4/1 -> Out5/1

== system SimulateHVDC/Subsystem ==
  Vc : Inport
  vB : Inport  Port=2
  MATLAB Function : MATLAB Function  TreatAsAtomicUnit=on
  vo_max : Outport
  vo_min : Outport  Port=2
  wires:
  MATLAB Function/1(vo_max) -> vo_max/1
  MATLAB Function/2(vo_min) -> vo_min/1
  Vc/1 -> MATLAB Function/1(Vc)
  vB/1 -> MATLAB Function/2(vB)

== system SimulateHVDC/Subsystem1 ==
  iB_ref : Inport
  MATLAB Function : MATLAB Function  TreatAsAtomicUnit=on  SystemSampleTime=CCMPC.Ts
  iz_max : Outport
  iz_min : Outport  Port=2
  wires:
  MATLAB Function/1(iz_max) -> iz_max/1
  MATLAB Function/2(iz_min) -> iz_min/1
  iB_ref/1 -> MATLAB Function/1(iB_ref)

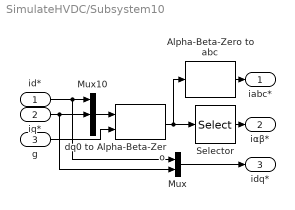
== system SimulateHVDC/Subsystem10 ==
  id* : Inport
  iq* : Inport  Port=2
  g : Inport  Port=3
  Alpha-Beta-Zero to abc : spsAlphaBetaZerotoabcLib/Alpha-Beta-Zero to abc
  Mux : Mux  Inputs=2
  Mux10 : Mux  Inputs=3
  Selector : Selector  InputPortWidth=3  IndexOptions=Index vector (dialog)  Indices=[1 2]  OutputSizes=1
  dq0 to Alpha-Beta-Zero : spsdq0toAlphaBetaZeroLib/dq0 to Alpha-Beta-Zero  Alignment=Aligned with phase A axis
  iabc* : Outport
  iαβ* : Outport  Port=2
  idq* : Outport  Port=3
  wires:
  dq0 to Alpha-Beta-Zero/1 -> Alpha-Beta-Zero to abc/1, Selector/1
  g/1 -> dq0 to Alpha-Beta-Zero/2
  Mux10/1 -> dq0 to Alpha-Beta-Zero/1
  Selector/1 -> iαβ*/1
  id*/1 -> Mux/1, Mux10/1
  Alpha-Beta-Zero to abc/1 -> iabc*/1
  iq*/1 -> Mux10/2, Mux/2
  Mux/1 -> idq*/1

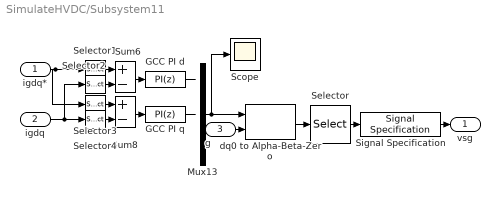
== system SimulateHVDC/Subsystem11 ==
  igdq* : Inport
  igdq : Inport  Port=2
  g : Inport  Port=3
  GCC PI d : slpidlib/PID Controller  Controller=PI  Form=Parallel  TimeDomain=Discrete-time  UseExternalTs=off  SampleTime=GCC.Ts  IntegratorMethod=Forward Euler  FilterMethod=Forward Euler  ControllerParametersSource=internal  P=GCC.kp  I=GCC.ki  UseKiTs=off  D=0  UseExternalDerivativeSource=off  N=100  UseFilter=on  TunerSelectOption=Transfer Function Based (PID Tuner App)  InitialConditionSource=internal  InitialConditionForIntegrator=0  InitialConditionForFilter=0  DifferentiatorICPrevScaledInput=0  ExternalReset=none  TrackingMode=off  Kt=1  LimitOutput=on  SatLimitsSource=internal  UpperSaturationLimit=M2C.Ay_max  LowerSaturationLimit=-M2C.Ay_max  LinearizeAsGain=on  AntiWindupMode=clamping  Kb=1  LimitIntegrator=off  UpperIntegratorSaturationLimit=inf  LowerIntegratorSaturationLimit=-inf  POutMin=[]  POutMax=[]  IOutMin=[]  IOutMax=[]  DOutMin=[]  DOutMax=[]  NOutMin=[]  NOutMax=[]  SumOutMin=[]  SumOutMax=[]  SaturationOutMin=[]  SaturationOutMax=[]  PParamMin=[]  PParamMax=[]  IParamMin=[]  IParamMax=[]  DParamMin=[]  DParamMax=[]  NParamMin=[]  NParamMax=[]  KbParamMin=[]  KbParamMax=[]  KtParamMin=[]  KtParamMax=[]  KbOutMin=[]  KbOutMax=[]  KtOutMin=[]  KtOutMax=[]  IntegratorOutMin=[]  IntegratorOutMax=[]  FilterOutMin=[]  FilterOutMax=[]  SumI1OutMin=[]  SumI1OutMax=[]  SumI2OutMin=[]  SumI2OutMax=[]  SumI3OutMin=[]  SumI3OutMax=[]  SumI4OutMin=[]  SumI4OutMax=[]  SumDOutMin=[]  SumDOutMax=[]  DifferentiatorOutMin=[]  DifferentiatorOutMax=[]  FilterDiffOutCoefMin=[]  FilterDiffOutCoefMax=[]  ReciprocalOutMin=[]  ReciprocalOutMax=[]  SumDenOutMin=[]  SumDenOutMax=[]  SumNumOutMin=[]  SumNumOutMax=[]  DivideOutMin=[]  DivideOutMax=[]  UdiffTsProdOutMin=[]  UdiffTsProdOutMax=[]  NTsProdOutMin=[]  NTsProdOutMax=[]  UintegralTsProdOutMin=[]  UintegralTsProdOutMax=[]  UngainTsProdOutMin=[]  UngainTsProdOutMax=[]  ClampingZeroOutDataTypeStr=Inherit: Inherit via back propagation  ClampingZeroOutMin=[]  ClampingZeroOutMax=[]  FilterDenConstantOutDataTypeStr=Inherit: Inherit via back propagation  FilterDenConstantOutMin=[]  FilterDenConstantOutMax=[]  PCopyOutDataTypeStr=Inherit: Inherit via back propagation  PCopyOutMin=[]  PCopyOutMax=[]  NCopyOutDataTypeStr=Inherit: Inherit via back propagation  NCopyOutMin=[]  NCopyOutMax=[]  IntegratorContinuousStateAttributes=''  IntegratorStateMustResolveToSignalObject=off  IntegratorRTWStateStorageClass=Auto  FilterContinuousStateAttributes=''  FilterStateMustResolveToSignalObject=off  FilterRTWStateStorageClass=Auto  ParallelPVariant=InternalParameters  IdealPVariant=Disabled  IVariant=InternalParameters  DVariant=Disabled  IntegratorVariant=Discrete  SatVariant=Enabled  AWVariant=DiscClampingParallel  PCopyVariant=Disabled  TRVariant=Disabled  FdbkBlocksVariant=Forward  IdealPFdbkVariant=Disabled  SatFdbkVariant=Disabled  DerivativeFilterVariant=Disabled  NVariant=Disabled  NCopyVariant=Disabled_SignalSpec  FilterICVariant=Disabled  IntegratorICVariant=InternalICs  ExternalResetVariant=Disabled  TRSumVariant=Passthrough  SumFdbkVariant=Disabled  SumVariant=Sum_PI  TsampFilterVariant=InternalTs  TsampNgainVariant=Passthrough  TsampIntegralVariant=Disabled_SignalSpec  ExternalSaturationOutDataTypeStr=Inherit: Same as second input  DerivativeSourceVariant=Disabled  PreIntVariant=InternalPreInt
  GCC PI q : slpidlib/PID Controller  Controller=PI  Form=Parallel  TimeDomain=Discrete-time  UseExternalTs=off  SampleTime=GCC.Ts  IntegratorMethod=Forward Euler  FilterMethod=Forward Euler  ControllerParametersSource=internal  P=GCC.kp  I=GCC.ki  UseKiTs=off  D=0  UseExternalDerivativeSource=off  N=100  UseFilter=on  TunerSelectOption=Transfer Function Based (PID Tuner App)  InitialConditionSource=internal  InitialConditionForIntegrator=0  InitialConditionForFilter=0  DifferentiatorICPrevScaledInput=0  ExternalReset=none  TrackingMode=off  Kt=1  LimitOutput=on  SatLimitsSource=internal  UpperSaturationLimit=M2C.Ay_max  LowerSaturationLimit=-M2C.Ay_max  LinearizeAsGain=on  AntiWindupMode=clamping  Kb=1  LimitIntegrator=off  UpperIntegratorSaturationLimit=inf  LowerIntegratorSaturationLimit=-inf  POutMin=[]  POutMax=[]  IOutMin=[]  IOutMax=[]  DOutMin=[]  DOutMax=[]  NOutMin=[]  NOutMax=[]  SumOutMin=[]  SumOutMax=[]  SaturationOutMin=[]  SaturationOutMax=[]  PParamMin=[]  PParamMax=[]  IParamMin=[]  IParamMax=[]  DParamMin=[]  DParamMax=[]  NParamMin=[]  NParamMax=[]  KbParamMin=[]  KbParamMax=[]  KtParamMin=[]  KtParamMax=[]  KbOutMin=[]  KbOutMax=[]  KtOutMin=[]  KtOutMax=[]  IntegratorOutMin=[]  IntegratorOutMax=[]  FilterOutMin=[]  FilterOutMax=[]  SumI1OutMin=[]  SumI1OutMax=[]  SumI2OutMin=[]  SumI2OutMax=[]  SumI3OutMin=[]  SumI3OutMax=[]  SumI4OutMin=[]  SumI4OutMax=[]  SumDOutMin=[]  SumDOutMax=[]  DifferentiatorOutMin=[]  DifferentiatorOutMax=[]  FilterDiffOutCoefMin=[]  FilterDiffOutCoefMax=[]  ReciprocalOutMin=[]  ReciprocalOutMax=[]  SumDenOutMin=[]  SumDenOutMax=[]  SumNumOutMin=[]  SumNumOutMax=[]  DivideOutMin=[]  DivideOutMax=[]  UdiffTsProdOutMin=[]  UdiffTsProdOutMax=[]  NTsProdOutMin=[]  NTsProdOutMax=[]  UintegralTsProdOutMin=[]  UintegralTsProdOutMax=[]  UngainTsProdOutMin=[]  UngainTsProdOutMax=[]  ClampingZeroOutDataTypeStr=Inherit: Inherit via back propagation  ClampingZeroOutMin=[]  ClampingZeroOutMax=[]  FilterDenConstantOutDataTypeStr=Inherit: Inherit via back propagation  FilterDenConstantOutMin=[]  FilterDenConstantOutMax=[]  PCopyOutDataTypeStr=Inherit: Inherit via back propagation  PCopyOutMin=[]  PCopyOutMax=[]  NCopyOutDataTypeStr=Inherit: Inherit via back propagation  NCopyOutMin=[]  NCopyOutMax=[]  IntegratorContinuousStateAttributes=''  IntegratorStateMustResolveToSignalObject=off  IntegratorRTWStateStorageClass=Auto  FilterContinuousStateAttributes=''  FilterStateMustResolveToSignalObject=off  FilterRTWStateStorageClass=Auto  ParallelPVariant=InternalParameters  IdealPVariant=Disabled  IVariant=InternalParameters  DVariant=Disabled  IntegratorVariant=Discrete  SatVariant=Enabled  AWVariant=DiscClampingParallel  PCopyVariant=Disabled  TRVariant=Disabled  FdbkBlocksVariant=Forward  IdealPFdbkVariant=Disabled  SatFdbkVariant=Disabled  DerivativeFilterVariant=Disabled  NVariant=Disabled  NCopyVariant=Disabled_SignalSpec  FilterICVariant=Disabled  IntegratorICVariant=InternalICs  ExternalResetVariant=Disabled  TRSumVariant=Passthrough  SumFdbkVariant=Disabled  SumVariant=Sum_PI  TsampFilterVariant=InternalTs  TsampNgainVariant=Passthrough  TsampIntegralVariant=Disabled_SignalSpec  ExternalSaturationOutDataTypeStr=Inherit: Same as second input  DerivativeSourceVariant=Disabled  PreIntVariant=InternalPreInt
  Mux13 : Mux  Inputs=3
  Scope : Scope
  Selector : Selector  InputPortWidth=3  IndexOptions=Index vector (dialog)  Indices=[1 2]  OutputSizes=1
  Selector1 : Selector  InputPortWidth=2  IndexOptions=Index vector (dialog)  Indices=[1]  OutputSizes=1
  Selector2 : Selector  InputPortWidth=2  IndexOptions=Index vector (dialog)  Indices=[1]  OutputSizes=1
  Selector3 : Selector  InputPortWidth=2  IndexOptions=Index vector (dialog)  Indices=[2]  OutputSizes=1
  Selector4 : Selector  InputPortWidth=2  IndexOptions=Index vector (dialog)  Indices=[2]  OutputSizes=1
  Signal Specification : SignalSpecification  Dimensions=[2, 1]  SampleTime=Ts_cc
  Sum6 : Sum  Inputs=+-
  Sum8 : Sum  Inputs=+-
  dq0 to Alpha-Beta-Zero : spsdq0toAlphaBetaZeroLib/dq0 to Alpha-Beta-Zero  Alignment=90 degrees behind phase A axis
  vsg : Outport
  wires:
  Selector2/1 -> Sum6/2
  Sum8/1 -> GCC PI q/1
  Selector3/1 -> Sum8/1
  Selector4/1 -> Sum8/2
  GCC PI q/1 -> ?
  Selector1/1 -> Sum6/1
  Sum6/1 -> GCC PI d/1
  GCC PI d/1 -> ?
  igdq*/1 -> Selector3/1, Selector1/1
  igdq/1 -> Selector2/1, Selector4/1
  Signal Specification/1 -> vsg/1
  Mux13/1 -> Scope/1, dq0 to Alpha-Beta-Zero/1
  g/1 -> dq0 to Alpha-Beta-Zero/2
  Selector/1 -> Signal Specification/1
  dq0 to Alpha-Beta-Zero/1 -> Selector/1

== system SimulateHVDC/Subsystem12 ==
  vx : Inport
  vg : Inport  Port=2
  Gain2 : Gain  Gain=M2C.A'  Multiplication=Matrix(K*u)
  Gain5 : Gain  Gain=[1, -1]  Multiplication=Matrix(K*u)
  Mux : Mux  Inputs=[2; 3]
  Vdc : Outport
  vxy : Outport  Port=2
  vB : Outport  Port=3
  wires:
  Mux/1 -> Gain2/1, vxy/1
  vx/1 -> Gain5/1, Mux/1
  Gain2/1 -> vB/1
  vg/1 -> Mux/2
  Gain5/1 -> Vdc/1

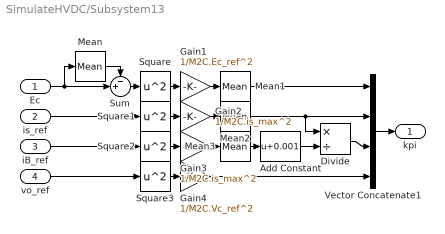
== system SimulateHVDC/Subsystem13 ==
  Ec : Inport
  is_ref : Inport  Port=2
  iB_ref : Inport  Port=3
  vo_ref : Inport  Port=4
  Add Constant : Bias  Bias=0.001  SaturateOnIntegerOverflow=off
  Divide : Product  Inputs=*/
  Gain1 : Gain  Gain=1/M2C.Ec_ref^2
  Gain2 : Gain  Gain=1/M2C.is_max^2
  Gain3 : Gain  Gain=1/M2C.is_max^2
  Gain4 : Gain  Gain=1/M2C.Vc_ref^2
  Mean{,1..3} (4 alike) : dspstat3/Mean  run=off  InputProcessing=Columns as channels (frame based)  reset_popup=None  directionMode=Entire input  dimension=1  roiEnable=off  roiType=Rectangles  roiPortion=Entire ROI  roiOutput=Individual statistics for each ROI  roiFlag=off  roundingMode=Floor  overflowMode=off  outputDataTypeStr=Inherit: Same as accumulator  outputMin=[]  outputMax=[]  outputLastDataTypeStr=Inherit: Same as accumulator
  Square{,1..3} (4 alike) : Math  Operator=square
  Sum : Sum  Inputs=-+|
  Vector Concatenate1 : Concatenate  NumInputs=4
  kpi : Outport
  wires:
  Mean1/1 -> Vector Concatenate1/1
  Square2/1 -> Gain3/1
  Gain3/1 -> Mean3/1
  Square3/1 -> Gain4/1
  Square/1 -> Gain1/1
  Add Constant/1 -> Divide/2
  Gain2/1 -> Mean2/1
  Gain1/1 -> Mean1/1
  Mean3/1 -> Add Constant/1
  Mean2/1 -> Vector Concatenate1/2, Divide/1
  is_ref/1 -> Square1/1
  Sum/1 -> Square/1
  Square1/1 -> Gain2/1
  Ec/1 -> Sum/2, Mean/1
  Mean/1 -> Sum/1
  Gain4/1 -> Vector Concatenate1/4
  Divide/1 -> Vector Concatenate1/3
  iB_ref/1 -> Square2/1
  Vector Concatenate1/1 -> kpi/1
  vo_ref/1 -> Square3/1

== system SimulateHVDC/Subsystem2 ==
  Vc : Inport
  MATLAB Function : MATLAB Function  TreatAsAtomicUnit=on  SystemSampleTime=CCMPC.Ts
  vs_max : Outport
  vs_min : Outport  Port=2
  wires:
  MATLAB Function/2(vs_min) -> vs_min/1
  Vc/1 -> MATLAB Function/1(Vc)
  MATLAB Function/1(vs_max) -> vs_max/1

== system SimulateHVDC/Subsystem3 ==
  is : Inport
  Gain1 : Gain  Gain=M2C.A  Multiplication=Matrix(K*u) (u vector)
  Gain3 : Gain  Gain=M2C.pinvA  Multiplication=Matrix(K*u) (u vector)
  Gain4 : Gain  Gain=M2C.pinvN  Multiplication=Matrix(K*u) (u vector)
  Sum3 : Sum  Inputs=-+|
  ixy : Outport
  iB : Outport  Port=2
  iz : Outport  Port=3
  ie : Outport  Port=4
  wires:
  Gain3/1 -> iB/1, Sum3/1
  is/1 -> Sum3/2, Gain1/1
  Gain1/1 -> ixy/1, Gain3/1
  Sum3/1 -> iz/1, Gain4/1
  Gain4/1 -> ie/1

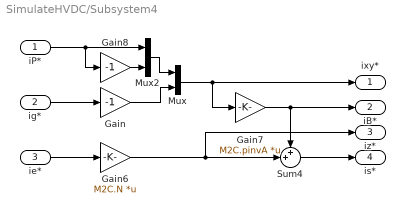
== system SimulateHVDC/Subsystem4 ==
  iP* : Inport
  ig* : Inport  Port=2
  ie* : Inport  Port=3
  Gain : Gain  Gain=-1
  Gain6 : Gain  Gain=M2C.N  Multiplication=Matrix(K*u)
  Gain7 : Gain  Gain=M2C.pinvA  Multiplication=Matrix(K*u)
  Gain8 : Gain  Gain=-1
  Mux : Mux  Inputs=[M2C.p; M2C.q]
  Mux2 : Mux  Inputs=2
  Sum4 : Sum  Inputs=++|
  ixy* : Outport
  iB* : Outport  Port=2
  iz* : Outport  Port=3
  is* : Outport  Port=4
  wires:
  ig*/1 -> Gain/1
  Mux2/1 -> Mux/1
  Gain8/1 -> Mux2/2
  iP*/1 -> Mux2/1, Gain8/1
  Gain/1 -> Mux/2
  Mux/1 -> Gain7/1, ixy*/1
  ie*/1 -> Gain6/1
  Sum4/1 -> is*/1
  Gain7/1 -> Sum4/1, iB*/1
  Gain6/1 -> iz*/1, Sum4/2

== system SimulateHVDC/Subsystem6 ==
  iP* : Inport
  iP : Inport  Port=2
  Constant1 : Constant  Value=3/2*M2C.Vdc  SampleTime=Ts_cc
  PCC PI : slpidlib/PID Controller  Controller=PI  Form=Parallel  TimeDomain=Discrete-time  UseExternalTs=off  SampleTime=PCC.Ts  IntegratorMethod=Forward Euler  FilterMethod=Forward Euler  ControllerParametersSource=internal  P=PCC.kp  I=PCC.ki  UseKiTs=off  D=0  UseExternalDerivativeSource=off  N=100  UseFilter=on  TunerSelectOption=Transfer Function Based (PID Tuner App)  InitialConditionSource=internal  InitialConditionForIntegrator=0  InitialConditionForFilter=0  DifferentiatorICPrevScaledInput=0  ExternalReset=none  TrackingMode=off  Kt=1  LimitOutput=on  SatLimitsSource=internal  UpperSaturationLimit=2 * M2C.Rb * M2C.ix_max  LowerSaturationLimit=-2 * M2C.Rb * M2C.ix_max  LinearizeAsGain=on  AntiWindupMode=clamping  Kb=1  LimitIntegrator=off  UpperIntegratorSaturationLimit=inf  LowerIntegratorSaturationLimit=-inf  POutMin=[]  POutMax=[]  IOutMin=[]  IOutMax=[]  DOutMin=[]  DOutMax=[]  NOutMin=[]  NOutMax=[]  SumOutMin=[]  SumOutMax=[]  SaturationOutMin=[]  SaturationOutMax=[]  PParamMin=[]  PParamMax=[]  IParamMin=[]  IParamMax=[]  DParamMin=[]  DParamMax=[]  NParamMin=[]  NParamMax=[]  KbParamMin=[]  KbParamMax=[]  KtParamMin=[]  KtParamMax=[]  KbOutMin=[]  KbOutMax=[]  KtOutMin=[]  KtOutMax=[]  IntegratorOutMin=[]  IntegratorOutMax=[]  FilterOutMin=[]  FilterOutMax=[]  SumI1OutMin=[]  SumI1OutMax=[]  SumI2OutMin=[]  SumI2OutMax=[]  SumI3OutMin=[]  SumI3OutMax=[]  SumI4OutMin=[]  SumI4OutMax=[]  SumDOutMin=[]  SumDOutMax=[]  DifferentiatorOutMin=[]  DifferentiatorOutMax=[]  FilterDiffOutCoefMin=[]  FilterDiffOutCoefMax=[]  ReciprocalOutMin=[]  ReciprocalOutMax=[]  SumDenOutMin=[]  SumDenOutMax=[]  SumNumOutMin=[]  SumNumOutMax=[]  DivideOutMin=[]  DivideOutMax=[]  UdiffTsProdOutMin=[]  UdiffTsProdOutMax=[]  NTsProdOutMin=[]  NTsProdOutMax=[]  UintegralTsProdOutMin=[]  UintegralTsProdOutMax=[]  UngainTsProdOutMin=[]  UngainTsProdOutMax=[]  ClampingZeroOutDataTypeStr=Inherit: Inherit via back propagation  ClampingZeroOutMin=[]  ClampingZeroOutMax=[]  FilterDenConstantOutDataTypeStr=Inherit: Inherit via back propagation  FilterDenConstantOutMin=[]  FilterDenConstantOutMax=[]  PCopyOutDataTypeStr=Inherit: Inherit via back propagation  PCopyOutMin=[]  PCopyOutMax=[]  NCopyOutDataTypeStr=Inherit: Inherit via back propagation  NCopyOutMin=[]  NCopyOutMax=[]  IntegratorContinuousStateAttributes=''  IntegratorStateMustResolveToSignalObject=off  IntegratorRTWStateStorageClass=Auto  FilterContinuousStateAttributes=''  FilterStateMustResolveToSignalObject=off  FilterRTWStateStorageClass=Auto  ParallelPVariant=InternalParameters  IdealPVariant=Disabled  IVariant=InternalParameters  DVariant=Disabled  IntegratorVariant=Discrete  SatVariant=Enabled  AWVariant=DiscClampingParallel  PCopyVariant=Disabled  TRVariant=Disabled  FdbkBlocksVariant=Forward  IdealPFdbkVariant=Disabled  SatFdbkVariant=Disabled  DerivativeFilterVariant=Disabled  NVariant=Disabled  NCopyVariant=Disabled_SignalSpec  FilterICVariant=Disabled  IntegratorICVariant=InternalICs  ExternalResetVariant=Disabled  TRSumVariant=Passthrough  SumFdbkVariant=Disabled  SumVariant=Sum_PI  TsampFilterVariant=InternalTs  TsampNgainVariant=Passthrough  TsampIntegralVariant=Disabled_SignalSpec  ExternalSaturationOutDataTypeStr=Inherit: Same as second input  DerivativeSourceVariant=Disabled  PreIntVariant=InternalPreInt
  Sum13 : Sum  Inputs=-+|
  Sum3 : Sum  Inputs=+-
  vsP : Outport
  wires:
  Sum3/1 -> PCC PI/1
  iP*/1 -> Sum3/1
  iP/1 -> Sum3/2
  Constant1/1 -> Sum13/1
  Sum13/1 -> vsP/1
  PCC PI/1 -> Sum13/2

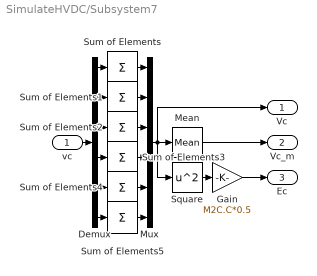
== system SimulateHVDC/Subsystem7 ==
  vc : Inport
  Demux : Demux  Outputs=[4; 4; 4; 4; 4; 4]
  Gain : Gain  Gain=M2C.C*0.5
  Mean : dspstat3/Mean  run=off  InputProcessing=Columns as channels (frame based)  reset_popup=None  directionMode=Entire input  dimension=1  roiEnable=off  roiType=Rectangles  roiPortion=Entire ROI  roiOutput=Individual statistics for each ROI  roiFlag=off  roundingMode=Floor  overflowMode=off  outputDataTypeStr=Inherit: Same as accumulator  outputMin=[]  outputMax=[]  outputLastDataTypeStr=Inherit: Same as accumulator
  Mux : Mux  Inputs=6
  Square : Math  Operator=square
  Sum of Elements{,1..5} (6 alike) : Sum  Inputs=+
  Vc : Outport
  Vc_m : Outport  Port=2
  Ec : Outport  Port=3
  wires:
  Square/1 -> Gain/1
  Gain/1 -> Ec/1
  Mean/1 -> Vc_m/1
  vc/1 -> Demux/1
  Demux/1 -> Sum of Elements/1
  Demux/2 -> Sum of Elements1/1
  Demux/3 -> Sum of Elements2/1
  Demux/4 -> Sum of Elements3/1
  Demux/5 -> Sum of Elements4/1
  Demux/6 -> Sum of Elements5/1
  Sum of Elements/1 -> Mux/1
  Sum of Elements1/1 -> Mux/2
  Sum of Elements2/1 -> Mux/3
  Sum of Elements3/1 -> Mux/4
  Sum of Elements4/1 -> Mux/5
  Sum of Elements5/1 -> Mux/6
  Mux/1 -> Vc/1, Square/1, Mean/1

== system SimulateHVDC/Subsystem8 ==
  vabc : Inport
  g : Inport  Port=2
  Alpha-Beta-Zero to dq0 : spsAlphaBetaZerotodq0Lib/Alpha-Beta-Zero to dq0  Alignment=90 degrees behind phase A axis
  Selector : Selector  InputPortWidth=3  IndexOptions=Index vector (dialog)  Indices=[1 2]  OutputSizes=1
  Selector1 : Selector  InputPortWidth=3  IndexOptions=Index vector (dialog)  Indices=[1 2]  OutputSizes=1
  abc to Alpha-Beta-Zero : spsabctoAlphaBetaZeroLib/abc to Alpha-Beta-Zero
  vαβ : Outport
  vdq : Outport  Port=2
  wires:
  vabc/1 -> abc to Alpha-Beta-Zero/1
  g/1 -> Alpha-Beta-Zero to dq0/2
  abc to Alpha-Beta-Zero/1 -> Selector/1, Alpha-Beta-Zero to dq0/1
  Selector/1 -> vαβ/1
  Alpha-Beta-Zero to dq0/1 -> Selector1/1
  Selector1/1 -> vdq/1

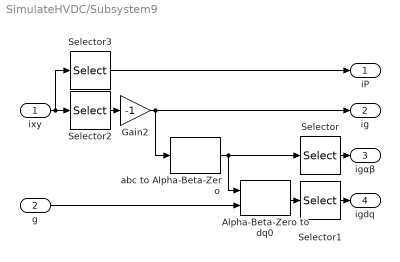
== system SimulateHVDC/Subsystem9 ==
  ixy : Inport
  g : Inport  Port=2
  Alpha-Beta-Zero to dq0 : spsAlphaBetaZerotodq0Lib/Alpha-Beta-Zero to dq0  Alignment=Aligned with phase A axis
  Gain2 : Gain  Gain=-1
  Selector : Selector  InputPortWidth=3  IndexOptions=Index vector (dialog)  Indices=[1 2]  OutputSizes=1
  Selector1 : Selector  InputPortWidth=3  IndexOptions=Index vector (dialog)  Indices=[1 2]  OutputSizes=1
  Selector2 : Selector  InputPortWidth=5  IndexOptions=Index vector (dialog)  Indices=[3 4 5]  OutputSizes=1
  Selector3 : Selector  InputPortWidth=5  IndexOptions=Index vector (dialog)  Indices=[1]  OutputSizes=1
  abc to Alpha-Beta-Zero : spsabctoAlphaBetaZeroLib/abc to Alpha-Beta-Zero
  iP : Outport
  ig : Outport  Port=2
  igαβ : Outport  Port=3
  igdq : Outport  Port=4
  wires:
  Selector/1 -> igαβ/1
  Alpha-Beta-Zero to dq0/1 -> Selector1/1
  abc to Alpha-Beta-Zero/1 -> Alpha-Beta-Zero to dq0/1, Selector/1
  g/1 -> Alpha-Beta-Zero to dq0/2
  ixy/1 -> Selector3/1, Selector2/1
  Selector1/1 -> igdq/1
  Gain2/1 -> ig/1, abc to Alpha-Beta-Zero/1
  Selector2/1 -> Gain2/1
  Selector3/1 -> iP/1

== system SimulateHVDC/M2C+HVDC/ CircuitID87  ==

== system SimulateHVDC/NN CEC/Subsystem ==
  input : Inport
  Trigger : TriggerPort  VariantControl=(inherit)  PortDimensions=1
  FFNN : deeplib/Predict  Network=Network from MAT-file  NetworkFunction=squeezenet  NetworkFilePath=F:\PabloJimenez\TESIS\ProyectoTesis\ProyectoTesis\ImitationLearningSimulink\ActualArchitecture\net.mat  MiniBatchSize=1  InputDataFormats={ 'input', 'CB' }  Predictions=on  Activations={}  ForceInterpretedSim=off  EnableDLNetwork=on  LastKnownNetworkFilePath='F:\PabloJimenez\TESIS\ProyectoTesis\ProyectoTesis\ImitationLearningSimulink\ActualArchitecture\net.mat'  LastKnownNetworkTimeStamp=739917.784224537084810435771942138671875
  output : Outport
  wires:
  input/1 -> FFNN/1
  FFNN/1 -> output/1

== matlab function SimulateHVDC/Subsystem1/MATLAB Function ==
  data: iB_ref input; iz_max output; M2C parameter; iz_min output
function [iz_max, iz_min] = iz_lim(iB_ref, M2C)
%#codegen

persistent is_max
if isempty(is_max)
    is_max = M2C.is_max;
end

iz_max = is_max - iB_ref;
iz_min = -is_max - iB_ref;

== matlab function SimulateHVDC/NN CEC/Reward function ==
  data: Ec input; is input; iB input; vo input; vB input; Vc input; r output; M2C parameter; IsDone output; UseExternalAction output; Ts_ce parameter
function [r, IsDone, UseExternalAction] = reward(Ec, is, iB, vo, vB, Vc, M2C, Ts_ce)
%#codegen

persistent Ec_ref Ec_ref2 Vc_ref2 is_max Vc_ref
if isempty(Ec_ref)
    Ec_ref  = M2C.Ec_ref;
    Ec_ref2 = Ec_ref;
    is_max = M2C.is_max;
    Vc_ref = M2C.Vc_ref;
    Vc_ref2 = Vc_ref^2;
end

% Penalize mean squared energy deviation
% r1>0, bigger as the deviation grows
r1 = 10*mean((Ec - mean(Ec)).^2) / Ec_ref2;

% Penalize deviation outside operative voltage
if or(min(Vc) < Vc_ref*0.85, Vc_ref*1.15 < max(Vc))
    r2 = 10;
    IsDone = true;
else
    r2 = 0;
    IsDone = false;
end

% Penalize circulating currents effect on resistive losses
% if iB=is, r3=0. if is>iB, r3>0;
r3 = max(min(mean(is.^2) / (mean(iB.^2) + 0.01) - 1, 1), 0);

% Penalize current limits
if any(is_max < abs(is))
    r4 = 1;
else
    r4 = 0;
end

% Penalize CMV
r5 = vo^2 / Vc_ref2;

% Penalize CMV limits
vo_max = min([Vc(1:3); zeros(3, 1)] - vB);
vo_min = max([zeros(3, 1); -Vc(4:6)] - vB);
if or(vo < vo_min, vo_max < vo)
    r6 = 1;
else
    r6 = 0;
end

% Use external action
% Penalize deviation outside operative voltage
if or(min(Vc) < Vc_ref*0.87, Vc_ref*1.13 < max(Vc))
    r7 = 10;
    UseExternalAction = true;
else
    r7 = 0;
    UseExternalAction = false;
end

% Total reward
r = -(r1 + r2 + r3 + r4 + r5 + r6 + r7) * Ts_ce;

== matlab function SimulateHVDC/Subsystem2/MATLAB Function ==
  data: Vc input; vs_max output; vs_min output
function [vs_max, vs_min] = vs_lim(Vc)

vs_max = [Vc(1:3); zeros(3, 1)];
vs_min = [zeros(3, 1); -Vc(4:6)];
